simulink model "w3_warplab_trigger_proc"  (Simulink 7.7)
settings: Solver=ode45  StartTime=0.0  StopTime=100  RelTol=1e-3
InitFcn:
  | warplab_trigger_proc_init
StartFcn:
  | warplab_trigger_proc_init
undefined symbols (not defined in the file or in its folder): gcbh, xlBlockLoadCallback, xlGetNormalizedPeriod
libraries: xbsIndex_r4 x817, xbsEDKLib_r4 x1
(part 4 of 6)

== system w3_warplab_trigger_proc/Registers/Input Configuration Slice2 ==
  32b : Inport
  (LSB+0):(LSB+4) : xbsIndex_r4/Slice  nbits=5  boolean_output=off  mode=Lower Bit Location + Width  bit1=0  base1=MSB of Input  bit0=0  base0=LSB of Input  dbl_ovrd=off  block_type=slice
  (LSB+16):(LSB+20) : xbsIndex_r4/Slice  nbits=5  boolean_output=off  mode=Lower Bit Location + Width  bit1=0  base1=MSB of Input  bit0=16  base0=LSB of Input  dbl_ovrd=off  block_type=slice
  (LSB+24):(LSB+28) : xbsIndex_r4/Slice  nbits=5  boolean_output=off  mode=Lower Bit Location + Width  bit1=0  base1=MSB of Input  bit0=24  base0=LSB of Input  dbl_ovrd=off  block_type=slice
  (LSB+8):(LSB+12) : xbsIndex_r4/Slice  nbits=5  boolean_output=off  mode=Lower Bit Location + Width  bit1=0  base1=MSB of Input  bit0=8  base0=LSB of Input  dbl_ovrd=off  block_type=slice
  LSB+13 : xbsIndex_r4/Slice  nbits=1  boolean_output=off  mode=Lower Bit Location + Width  bit1=0  base1=MSB of Input  bit0=13  base0=LSB of Input  dbl_ovrd=off  block_type=slice
  LSB+14 : xbsIndex_r4/Slice  nbits=1  boolean_output=off  mode=Lower Bit Location + Width  bit1=0  base1=MSB of Input  bit0=14  base0=LSB of Input  dbl_ovrd=off  block_type=slice
  LSB+21 : xbsIndex_r4/Slice  nbits=1  boolean_output=off  mode=Lower Bit Location + Width  bit1=0  base1=MSB of Input  bit0=21  base0=LSB of Input  dbl_ovrd=off  block_type=slice
  LSB+22 : xbsIndex_r4/Slice  nbits=1  boolean_output=off  mode=Lower Bit Location + Width  bit1=0  base1=MSB of Input  bit0=22  base0=LSB of Input  dbl_ovrd=off  block_type=slice
  LSB+29 : xbsIndex_r4/Slice  nbits=1  boolean_output=off  mode=Lower Bit Location + Width  bit1=0  base1=MSB of Input  bit0=29  base0=LSB of Input  dbl_ovrd=off  block_type=slice
  LSB+31 : xbsIndex_r4/Slice  nbits=1  boolean_output=off  mode=Lower Bit Location + Width  bit1=0  base1=MSB of Input  bit0=31  base0=LSB of Input  dbl_ovrd=off  block_type=slice
  LSB+5 : xbsIndex_r4/Slice  nbits=1  boolean_output=off  mode=Lower Bit Location + Width  bit1=0  base1=MSB of Input  bit0=5  base0=LSB of Input  dbl_ovrd=off  block_type=slice
  LSB+6 : xbsIndex_r4/Slice  nbits=1  boolean_output=off  mode=Lower Bit Location + Width  bit1=0  base1=MSB of Input  bit0=6  base0=LSB of Input  dbl_ovrd=off  block_type=slice
  Delay 1 : Outport
  Debounce 1 : Outport  Port=2
  Reset 1 : Outport  Port=3
  Delay 2 : Outport  Port=4
  Debounce 2 : Outport  Port=5
  Reset 2 : Outport  Port=6
  Delay 3 : Outport  Port=7
  Debounce 3 : Outport  Port=8
  Reset 3 : Outport  Port=9
  Delay 4 : Outport  Port=10
  Soft Trig : Outport  Port=11
  Reset 4 : Outport  Port=12
  wires:
  LSB+31/1 -> Reset 4/1
  LSB+29/1 -> Soft Trig/1
  (LSB+24):(LSB+28)/1 -> Delay 4/1
  LSB+22/1 -> Reset 3/1
  LSB+21/1 -> Debounce 3/1
  (LSB+16):(LSB+20)/1 -> Delay 3/1
  LSB+14/1 -> Reset 2/1
  LSB+13/1 -> Debounce 2/1
  (LSB+8):(LSB+12)/1 -> Delay 2/1
  LSB+6/1 -> Reset 1/1
  LSB+5/1 -> Debounce 1/1
  (LSB+0):(LSB+4)/1 -> Delay 1/1
  32b/1 -> (LSB+0):(LSB+4)/1, LSB+5/1, LSB+6/1, (LSB+8):(LSB+12)/1, LSB+13/1, LSB+14/1, (LSB+16):(LSB+20)/1, LSB+21/1, LSB+22/1, (LSB+24):(LSB+28)/1, LSB+29/1, LSB+31/1

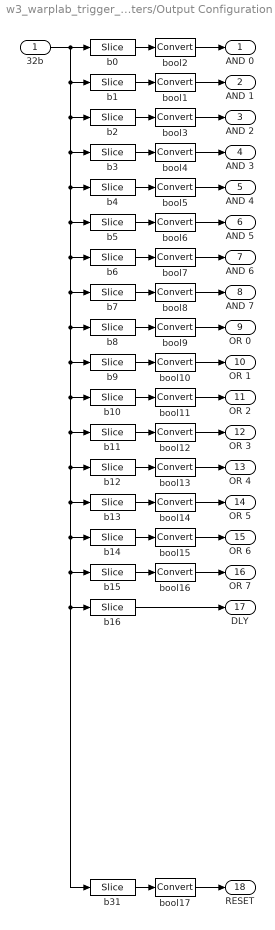
== system w3_warplab_trigger_proc/Registers/Output Configuration Slice ==
  32b : Inport
  b0 : xbsIndex_r4/Slice  nbits=1  boolean_output=off  mode=Lower Bit Location + Width  bit1=0  base1=MSB of Input  bit0=0  base0=LSB of Input  dbl_ovrd=off  block_type=slice
  b1 : xbsIndex_r4/Slice  nbits=1  boolean_output=off  mode=Lower Bit Location + Width  bit1=0  base1=MSB of Input  bit0=1  base0=LSB of Input  dbl_ovrd=off  block_type=slice
  b10 : xbsIndex_r4/Slice  nbits=1  boolean_output=off  mode=Lower Bit Location + Width  bit1=0  base1=MSB of Input  bit0=10  base0=LSB of Input  dbl_ovrd=off  block_type=slice
  b11 : xbsIndex_r4/Slice  nbits=1  boolean_output=off  mode=Lower Bit Location + Width  bit1=0  base1=MSB of Input  bit0=11  base0=LSB of Input  dbl_ovrd=off  block_type=slice
  b12 : xbsIndex_r4/Slice  nbits=1  boolean_output=off  mode=Lower Bit Location + Width  bit1=0  base1=MSB of Input  bit0=12  base0=LSB of Input  dbl_ovrd=off  block_type=slice
  b13 : xbsIndex_r4/Slice  nbits=1  boolean_output=off  mode=Lower Bit Location + Width  bit1=0  base1=MSB of Input  bit0=13  base0=LSB of Input  dbl_ovrd=off  block_type=slice
  b14 : xbsIndex_r4/Slice  nbits=1  boolean_output=off  mode=Lower Bit Location + Width  bit1=0  base1=MSB of Input  bit0=14  base0=LSB of Input  dbl_ovrd=off  block_type=slice
  b15 : xbsIndex_r4/Slice  nbits=1  boolean_output=off  mode=Lower Bit Location + Width  bit1=0  base1=MSB of Input  bit0=15  base0=LSB of Input  dbl_ovrd=off  block_type=slice
  b16 : xbsIndex_r4/Slice  nbits=5  boolean_output=off  mode=Lower Bit Location + Width  bit1=0  base1=MSB of Input  bit0=16  base0=LSB of Input  dbl_ovrd=off  block_type=slice
  b2 : xbsIndex_r4/Slice  nbits=1  boolean_output=off  mode=Lower Bit Location + Width  bit1=0  base1=MSB of Input  bit0=2  base0=LSB of Input  dbl_ovrd=off  block_type=slice
  b3 : xbsIndex_r4/Slice  nbits=1  boolean_output=off  mode=Lower Bit Location + Width  bit1=0  base1=MSB of Input  bit0=3  base0=LSB of Input  dbl_ovrd=off  block_type=slice
  b31 : xbsIndex_r4/Slice  nbits=1  boolean_output=off  mode=Lower Bit Location + Width  bit1=0  base1=MSB of Input  bit0=31  base0=LSB of Input  dbl_ovrd=off  block_type=slice
  b4 : xbsIndex_r4/Slice  nbits=1  boolean_output=off  mode=Lower Bit Location + Width  bit1=0  base1=MSB of Input  bit0=4  base0=LSB of Input  dbl_ovrd=off  block_type=slice
  b5 : xbsIndex_r4/Slice  nbits=1  boolean_output=off  mode=Lower Bit Location + Width  bit1=0  base1=MSB of Input  bit0=5  base0=LSB of Input  dbl_ovrd=off  block_type=slice
  b6 : xbsIndex_r4/Slice  nbits=1  boolean_output=off  mode=Lower Bit Location + Width  bit1=0  base1=MSB of Input  bit0=6  base0=LSB of Input  dbl_ovrd=off  block_type=slice
  b7 : xbsIndex_r4/Slice  nbits=1  boolean_output=off  mode=Lower Bit Location + Width  bit1=0  base1=MSB of Input  bit0=7  base0=LSB of Input  dbl_ovrd=off  block_type=slice
  b8 : xbsIndex_r4/Slice  nbits=1  boolean_output=off  mode=Lower Bit Location + Width  bit1=0  base1=MSB of Input  bit0=8  base0=LSB of Input  dbl_ovrd=off  block_type=slice
  b9 : xbsIndex_r4/Slice  nbits=1  boolean_output=off  mode=Lower Bit Location + Width  bit1=0  base1=MSB of Input  bit0=9  base0=LSB of Input  dbl_ovrd=off  block_type=slice
  bool{1..17} (17 alike) : xbsIndex_r4/Convert  gui_display_data_type=Boolean  arith_type=Boolean  n_bits=16  bin_pt=14  float_type=Single  exp_bits=8  fraction_bits=24  quantization=Truncate  overflow=Wrap  en=off  latency=0  dbl_ovrd=off  pipeline=off  block_type=convert
  AND 0 : Outport
  AND 1 : Outport  Port=2
  AND 2 : Outport  Port=3
  AND 3 : Outport  Port=4
  AND 4 : Outport  Port=5
  AND 5 : Outport  Port=6
  AND 6 : Outport  Port=7
  AND 7 : Outport  Port=8
  OR 0 : Outport  Port=9
  OR 1 : Outport  Port=10
  OR 2 : Outport  Port=11
  OR 3 : Outport  Port=12
  OR 4 : Outport  Port=13
  OR 5 : Outport  Port=14
  OR 6 : Outport  Port=15
  OR 7 : Outport  Port=16
  DLY : Outport  Port=17
  RESET : Outport  Port=18
  wires:
  32b/1 -> b0/1, b1/1, b2/1, b3/1, b4/1, b5/1, b6/1, b7/1, b8/1, b9/1, b10/1, b11/1, b12/1, b13/1, b14/1, b15/1, b31/1, b16/1
  b0/1 -> bool2/1
  b1/1 -> bool1/1
  b2/1 -> bool3/1
  b3/1 -> bool4/1
  b4/1 -> bool5/1
  b5/1 -> bool6/1
  b6/1 -> bool7/1
  b7/1 -> bool8/1
  b8/1 -> bool9/1
  b9/1 -> bool10/1
  b10/1 -> bool11/1
  b11/1 -> bool12/1
  b12/1 -> bool13/1
  b13/1 -> bool14/1
  b14/1 -> bool15/1
  b31/1 -> bool17/1
  b15/1 -> bool16/1
  bool2/1 -> AND 0/1
  bool1/1 -> AND 1/1
  bool3/1 -> AND 2/1
  bool4/1 -> AND 3/1
  bool5/1 -> AND 4/1
  bool6/1 -> AND 5/1
  bool7/1 -> AND 6/1
  bool8/1 -> AND 7/1
  bool9/1 -> OR 0/1
  bool10/1 -> OR 1/1
  bool11/1 -> OR 2/1
  bool12/1 -> OR 3/1
  bool13/1 -> OR 4/1
  bool14/1 -> OR 5/1
  bool15/1 -> OR 6/1
  bool16/1 -> OR 7/1
  bool17/1 -> RESET/1
  b16/1 -> DLY/1

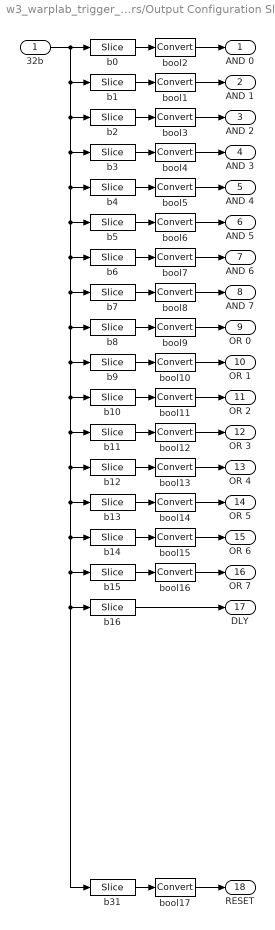
== system w3_warplab_trigger_proc/Registers/Output Configuration Slice1 ==
  32b : Inport
  b0 : xbsIndex_r4/Slice  nbits=1  boolean_output=off  mode=Lower Bit Location + Width  bit1=0  base1=MSB of Input  bit0=0  base0=LSB of Input  dbl_ovrd=off  block_type=slice
  b1 : xbsIndex_r4/Slice  nbits=1  boolean_output=off  mode=Lower Bit Location + Width  bit1=0  base1=MSB of Input  bit0=1  base0=LSB of Input  dbl_ovrd=off  block_type=slice
  b10 : xbsIndex_r4/Slice  nbits=1  boolean_output=off  mode=Lower Bit Location + Width  bit1=0  base1=MSB of Input  bit0=10  base0=LSB of Input  dbl_ovrd=off  block_type=slice
  b11 : xbsIndex_r4/Slice  nbits=1  boolean_output=off  mode=Lower Bit Location + Width  bit1=0  base1=MSB of Input  bit0=11  base0=LSB of Input  dbl_ovrd=off  block_type=slice
  b12 : xbsIndex_r4/Slice  nbits=1  boolean_output=off  mode=Lower Bit Location + Width  bit1=0  base1=MSB of Input  bit0=12  base0=LSB of Input  dbl_ovrd=off  block_type=slice
  b13 : xbsIndex_r4/Slice  nbits=1  boolean_output=off  mode=Lower Bit Location + Width  bit1=0  base1=MSB of Input  bit0=13  base0=LSB of Input  dbl_ovrd=off  block_type=slice
  b14 : xbsIndex_r4/Slice  nbits=1  boolean_output=off  mode=Lower Bit Location + Width  bit1=0  base1=MSB of Input  bit0=14  base0=LSB of Input  dbl_ovrd=off  block_type=slice
  b15 : xbsIndex_r4/Slice  nbits=1  boolean_output=off  mode=Lower Bit Location + Width  bit1=0  base1=MSB of Input  bit0=15  base0=LSB of Input  dbl_ovrd=off  block_type=slice
  b16 : xbsIndex_r4/Slice  nbits=5  boolean_output=off  mode=Lower Bit Location + Width  bit1=0  base1=MSB of Input  bit0=16  base0=LSB of Input  dbl_ovrd=off  block_type=slice
  b2 : xbsIndex_r4/Slice  nbits=1  boolean_output=off  mode=Lower Bit Location + Width  bit1=0  base1=MSB of Input  bit0=2  base0=LSB of Input  dbl_ovrd=off  block_type=slice
  b3 : xbsIndex_r4/Slice  nbits=1  boolean_output=off  mode=Lower Bit Location + Width  bit1=0  base1=MSB of Input  bit0=3  base0=LSB of Input  dbl_ovrd=off  block_type=slice
  b31 : xbsIndex_r4/Slice  nbits=1  boolean_output=off  mode=Lower Bit Location + Width  bit1=0  base1=MSB of Input  bit0=31  base0=LSB of Input  dbl_ovrd=off  block_type=slice
  b4 : xbsIndex_r4/Slice  nbits=1  boolean_output=off  mode=Lower Bit Location + Width  bit1=0  base1=MSB of Input  bit0=4  base0=LSB of Input  dbl_ovrd=off  block_type=slice
  b5 : xbsIndex_r4/Slice  nbits=1  boolean_output=off  mode=Lower Bit Location + Width  bit1=0  base1=MSB of Input  bit0=5  base0=LSB of Input  dbl_ovrd=off  block_type=slice
  b6 : xbsIndex_r4/Slice  nbits=1  boolean_output=off  mode=Lower Bit Location + Width  bit1=0  base1=MSB of Input  bit0=6  base0=LSB of Input  dbl_ovrd=off  block_type=slice
  b7 : xbsIndex_r4/Slice  nbits=1  boolean_output=off  mode=Lower Bit Location + Width  bit1=0  base1=MSB of Input  bit0=7  base0=LSB of Input  dbl_ovrd=off  block_type=slice
  b8 : xbsIndex_r4/Slice  nbits=1  boolean_output=off  mode=Lower Bit Location + Width  bit1=0  base1=MSB of Input  bit0=8  base0=LSB of Input  dbl_ovrd=off  block_type=slice
  b9 : xbsIndex_r4/Slice  nbits=1  boolean_output=off  mode=Lower Bit Location + Width  bit1=0  base1=MSB of Input  bit0=9  base0=LSB of Input  dbl_ovrd=off  block_type=slice
  bool{1..17} (17 alike) : xbsIndex_r4/Convert  gui_display_data_type=Boolean  arith_type=Boolean  n_bits=16  bin_pt=14  float_type=Single  exp_bits=8  fraction_bits=24  quantization=Truncate  overflow=Wrap  en=off  latency=0  dbl_ovrd=off  pipeline=off  block_type=convert
  AND 0 : Outport
  AND 1 : Outport  Port=2
  AND 2 : Outport  Port=3
  AND 3 : Outport  Port=4
  AND 4 : Outport  Port=5
  AND 5 : Outport  Port=6
  AND 6 : Outport  Port=7
  AND 7 : Outport  Port=8
  OR 0 : Outport  Port=9
  OR 1 : Outport  Port=10
  OR 2 : Outport  Port=11
  OR 3 : Outport  Port=12
  OR 4 : Outport  Port=13
  OR 5 : Outport  Port=14
  OR 6 : Outport  Port=15
  OR 7 : Outport  Port=16
  DLY : Outport  Port=17
  RESET : Outport  Port=18
  wires:
  b16/1 -> DLY/1
  bool17/1 -> RESET/1
  bool16/1 -> OR 7/1
  bool15/1 -> OR 6/1
  bool14/1 -> OR 5/1
  bool13/1 -> OR 4/1
  bool12/1 -> OR 3/1
  bool11/1 -> OR 2/1
  bool10/1 -> OR 1/1
  bool9/1 -> OR 0/1
  bool8/1 -> AND 7/1
  bool7/1 -> AND 6/1
  bool6/1 -> AND 5/1
  bool5/1 -> AND 4/1
  bool4/1 -> AND 3/1
  bool3/1 -> AND 2/1
  bool1/1 -> AND 1/1
  bool2/1 -> AND 0/1
  b15/1 -> bool16/1
  b31/1 -> bool17/1
  b14/1 -> bool15/1
  b13/1 -> bool14/1
  b12/1 -> bool13/1
  b11/1 -> bool12/1
  b10/1 -> bool11/1
  b9/1 -> bool10/1
  b8/1 -> bool9/1
  b7/1 -> bool8/1
  b6/1 -> bool7/1
  b5/1 -> bool6/1
  b4/1 -> bool5/1
  b3/1 -> bool4/1
  b2/1 -> bool3/1
  b1/1 -> bool1/1
  b0/1 -> bool2/1
  32b/1 -> b16/1, b31/1, b15/1, b14/1, b13/1, b12/1, b11/1, b10/1, b9/1, b8/1, b7/1, b6/1, b5/1, b4/1, b3/1, b2/1, b1/1, b0/1

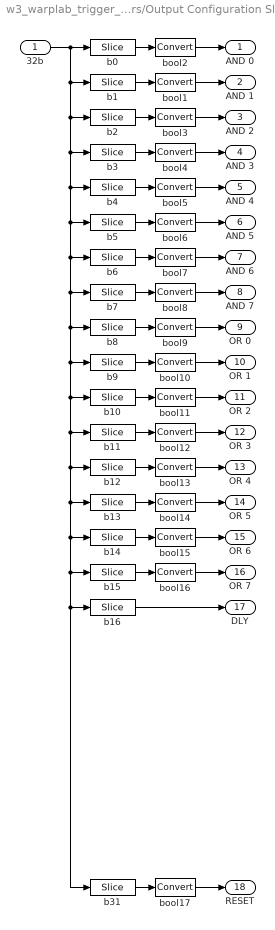
== system w3_warplab_trigger_proc/Registers/Output Configuration Slice2 ==
  32b : Inport
  b0 : xbsIndex_r4/Slice  nbits=1  boolean_output=off  mode=Lower Bit Location + Width  bit1=0  base1=MSB of Input  bit0=0  base0=LSB of Input  dbl_ovrd=off  block_type=slice
  b1 : xbsIndex_r4/Slice  nbits=1  boolean_output=off  mode=Lower Bit Location + Width  bit1=0  base1=MSB of Input  bit0=1  base0=LSB of Input  dbl_ovrd=off  block_type=slice
  b10 : xbsIndex_r4/Slice  nbits=1  boolean_output=off  mode=Lower Bit Location + Width  bit1=0  base1=MSB of Input  bit0=10  base0=LSB of Input  dbl_ovrd=off  block_type=slice
  b11 : xbsIndex_r4/Slice  nbits=1  boolean_output=off  mode=Lower Bit Location + Width  bit1=0  base1=MSB of Input  bit0=11  base0=LSB of Input  dbl_ovrd=off  block_type=slice
  b12 : xbsIndex_r4/Slice  nbits=1  boolean_output=off  mode=Lower Bit Location + Width  bit1=0  base1=MSB of Input  bit0=12  base0=LSB of Input  dbl_ovrd=off  block_type=slice
  b13 : xbsIndex_r4/Slice  nbits=1  boolean_output=off  mode=Lower Bit Location + Width  bit1=0  base1=MSB of Input  bit0=13  base0=LSB of Input  dbl_ovrd=off  block_type=slice
  b14 : xbsIndex_r4/Slice  nbits=1  boolean_output=off  mode=Lower Bit Location + Width  bit1=0  base1=MSB of Input  bit0=14  base0=LSB of Input  dbl_ovrd=off  block_type=slice
  b15 : xbsIndex_r4/Slice  nbits=1  boolean_output=off  mode=Lower Bit Location + Width  bit1=0  base1=MSB of Input  bit0=15  base0=LSB of Input  dbl_ovrd=off  block_type=slice
  b16 : xbsIndex_r4/Slice  nbits=5  boolean_output=off  mode=Lower Bit Location + Width  bit1=0  base1=MSB of Input  bit0=16  base0=LSB of Input  dbl_ovrd=off  block_type=slice
  b2 : xbsIndex_r4/Slice  nbits=1  boolean_output=off  mode=Lower Bit Location + Width  bit1=0  base1=MSB of Input  bit0=2  base0=LSB of Input  dbl_ovrd=off  block_type=slice
  b3 : xbsIndex_r4/Slice  nbits=1  boolean_output=off  mode=Lower Bit Location + Width  bit1=0  base1=MSB of Input  bit0=3  base0=LSB of Input  dbl_ovrd=off  block_type=slice
  b31 : xbsIndex_r4/Slice  nbits=1  boolean_output=off  mode=Lower Bit Location + Width  bit1=0  base1=MSB of Input  bit0=31  base0=LSB of Input  dbl_ovrd=off  block_type=slice
  b4 : xbsIndex_r4/Slice  nbits=1  boolean_output=off  mode=Lower Bit Location + Width  bit1=0  base1=MSB of Input  bit0=4  base0=LSB of Input  dbl_ovrd=off  block_type=slice
  b5 : xbsIndex_r4/Slice  nbits=1  boolean_output=off  mode=Lower Bit Location + Width  bit1=0  base1=MSB of Input  bit0=5  base0=LSB of Input  dbl_ovrd=off  block_type=slice
  b6 : xbsIndex_r4/Slice  nbits=1  boolean_output=off  mode=Lower Bit Location + Width  bit1=0  base1=MSB of Input  bit0=6  base0=LSB of Input  dbl_ovrd=off  block_type=slice
  b7 : xbsIndex_r4/Slice  nbits=1  boolean_output=off  mode=Lower Bit Location + Width  bit1=0  base1=MSB of Input  bit0=7  base0=LSB of Input  dbl_ovrd=off  block_type=slice
  b8 : xbsIndex_r4/Slice  nbits=1  boolean_output=off  mode=Lower Bit Location + Width  bit1=0  base1=MSB of Input  bit0=8  base0=LSB of Input  dbl_ovrd=off  block_type=slice
  b9 : xbsIndex_r4/Slice  nbits=1  boolean_output=off  mode=Lower Bit Location + Width  bit1=0  base1=MSB of Input  bit0=9  base0=LSB of Input  dbl_ovrd=off  block_type=slice
  bool{1..17} (17 alike) : xbsIndex_r4/Convert  gui_display_data_type=Boolean  arith_type=Boolean  n_bits=16  bin_pt=14  float_type=Single  exp_bits=8  fraction_bits=24  quantization=Truncate  overflow=Wrap  en=off  latency=0  dbl_ovrd=off  pipeline=off  block_type=convert
  AND 0 : Outport
  AND 1 : Outport  Port=2
  AND 2 : Outport  Port=3
  AND 3 : Outport  Port=4
  AND 4 : Outport  Port=5
  AND 5 : Outport  Port=6
  AND 6 : Outport  Port=7
  AND 7 : Outport  Port=8
  OR 0 : Outport  Port=9
  OR 1 : Outport  Port=10
  OR 2 : Outport  Port=11
  OR 3 : Outport  Port=12
  OR 4 : Outport  Port=13
  OR 5 : Outport  Port=14
  OR 6 : Outport  Port=15
  OR 7 : Outport  Port=16
  DLY : Outport  Port=17
  RESET : Outport  Port=18
  wires:
  32b/1 -> b0/1, b1/1, b2/1, b3/1, b4/1, b5/1, b6/1, b7/1, b8/1, b9/1, b10/1, b11/1, b12/1, b13/1, b14/1, b15/1, b31/1, b16/1
  b0/1 -> bool2/1
  b1/1 -> bool1/1
  b2/1 -> bool3/1
  b3/1 -> bool4/1
  b4/1 -> bool5/1
  b5/1 -> bool6/1
  b6/1 -> bool7/1
  b7/1 -> bool8/1
  b8/1 -> bool9/1
  b9/1 -> bool10/1
  b10/1 -> bool11/1
  b11/1 -> bool12/1
  b12/1 -> bool13/1
  b13/1 -> bool14/1
  b14/1 -> bool15/1
  b31/1 -> bool17/1
  b15/1 -> bool16/1
  bool2/1 -> AND 0/1
  bool1/1 -> AND 1/1
  bool3/1 -> AND 2/1
  bool4/1 -> AND 3/1
  bool5/1 -> AND 4/1
  bool6/1 -> AND 5/1
  bool7/1 -> AND 6/1
  bool8/1 -> AND 7/1
  bool9/1 -> OR 0/1
  bool10/1 -> OR 1/1
  bool11/1 -> OR 2/1
  bool12/1 -> OR 3/1
  bool13/1 -> OR 4/1
  bool14/1 -> OR 5/1
  bool15/1 -> OR 6/1
  bool16/1 -> OR 7/1
  bool17/1 -> RESET/1
  b16/1 -> DLY/1

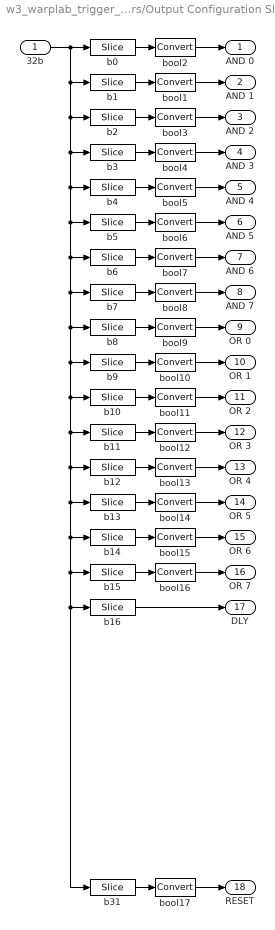
== system w3_warplab_trigger_proc/Registers/Output Configuration Slice3 ==
  32b : Inport
  b0 : xbsIndex_r4/Slice  nbits=1  boolean_output=off  mode=Lower Bit Location + Width  bit1=0  base1=MSB of Input  bit0=0  base0=LSB of Input  dbl_ovrd=off  block_type=slice
  b1 : xbsIndex_r4/Slice  nbits=1  boolean_output=off  mode=Lower Bit Location + Width  bit1=0  base1=MSB of Input  bit0=1  base0=LSB of Input  dbl_ovrd=off  block_type=slice
  b10 : xbsIndex_r4/Slice  nbits=1  boolean_output=off  mode=Lower Bit Location + Width  bit1=0  base1=MSB of Input  bit0=10  base0=LSB of Input  dbl_ovrd=off  block_type=slice
  b11 : xbsIndex_r4/Slice  nbits=1  boolean_output=off  mode=Lower Bit Location + Width  bit1=0  base1=MSB of Input  bit0=11  base0=LSB of Input  dbl_ovrd=off  block_type=slice
  b12 : xbsIndex_r4/Slice  nbits=1  boolean_output=off  mode=Lower Bit Location + Width  bit1=0  base1=MSB of Input  bit0=12  base0=LSB of Input  dbl_ovrd=off  block_type=slice
  b13 : xbsIndex_r4/Slice  nbits=1  boolean_output=off  mode=Lower Bit Location + Width  bit1=0  base1=MSB of Input  bit0=13  base0=LSB of Input  dbl_ovrd=off  block_type=slice
  b14 : xbsIndex_r4/Slice  nbits=1  boolean_output=off  mode=Lower Bit Location + Width  bit1=0  base1=MSB of Input  bit0=14  base0=LSB of Input  dbl_ovrd=off  block_type=slice
  b15 : xbsIndex_r4/Slice  nbits=1  boolean_output=off  mode=Lower Bit Location + Width  bit1=0  base1=MSB of Input  bit0=15  base0=LSB of Input  dbl_ovrd=off  block_type=slice
  b16 : xbsIndex_r4/Slice  nbits=5  boolean_output=off  mode=Lower Bit Location + Width  bit1=0  base1=MSB of Input  bit0=16  base0=LSB of Input  dbl_ovrd=off  block_type=slice
  b2 : xbsIndex_r4/Slice  nbits=1  boolean_output=off  mode=Lower Bit Location + Width  bit1=0  base1=MSB of Input  bit0=2  base0=LSB of Input  dbl_ovrd=off  block_type=slice
  b3 : xbsIndex_r4/Slice  nbits=1  boolean_output=off  mode=Lower Bit Location + Width  bit1=0  base1=MSB of Input  bit0=3  base0=LSB of Input  dbl_ovrd=off  block_type=slice
  b31 : xbsIndex_r4/Slice  nbits=1  boolean_output=off  mode=Lower Bit Location + Width  bit1=0  base1=MSB of Input  bit0=31  base0=LSB of Input  dbl_ovrd=off  block_type=slice
  b4 : xbsIndex_r4/Slice  nbits=1  boolean_output=off  mode=Lower Bit Location + Width  bit1=0  base1=MSB of Input  bit0=4  base0=LSB of Input  dbl_ovrd=off  block_type=slice
  b5 : xbsIndex_r4/Slice  nbits=1  boolean_output=off  mode=Lower Bit Location + Width  bit1=0  base1=MSB of Input  bit0=5  base0=LSB of Input  dbl_ovrd=off  block_type=slice
  b6 : xbsIndex_r4/Slice  nbits=1  boolean_output=off  mode=Lower Bit Location + Width  bit1=0  base1=MSB of Input  bit0=6  base0=LSB of Input  dbl_ovrd=off  block_type=slice
  b7 : xbsIndex_r4/Slice  nbits=1  boolean_output=off  mode=Lower Bit Location + Width  bit1=0  base1=MSB of Input  bit0=7  base0=LSB of Input  dbl_ovrd=off  block_type=slice
  b8 : xbsIndex_r4/Slice  nbits=1  boolean_output=off  mode=Lower Bit Location + Width  bit1=0  base1=MSB of Input  bit0=8  base0=LSB of Input  dbl_ovrd=off  block_type=slice
  b9 : xbsIndex_r4/Slice  nbits=1  boolean_output=off  mode=Lower Bit Location + Width  bit1=0  base1=MSB of Input  bit0=9  base0=LSB of Input  dbl_ovrd=off  block_type=slice
  bool{1..17} (17 alike) : xbsIndex_r4/Convert  gui_display_data_type=Boolean  arith_type=Boolean  n_bits=16  bin_pt=14  float_type=Single  exp_bits=8  fraction_bits=24  quantization=Truncate  overflow=Wrap  en=off  latency=0  dbl_ovrd=off  pipeline=off  block_type=convert
  AND 0 : Outport
  AND 1 : Outport  Port=2
  AND 2 : Outport  Port=3
  AND 3 : Outport  Port=4
  AND 4 : Outport  Port=5
  AND 5 : Outport  Port=6
  AND 6 : Outport  Port=7
  AND 7 : Outport  Port=8
  OR 0 : Outport  Port=9
  OR 1 : Outport  Port=10
  OR 2 : Outport  Port=11
  OR 3 : Outport  Port=12
  OR 4 : Outport  Port=13
  OR 5 : Outport  Port=14
  OR 6 : Outport  Port=15
  OR 7 : Outport  Port=16
  DLY : Outport  Port=17
  RESET : Outport  Port=18
  wires:
  b16/1 -> DLY/1
  bool17/1 -> RESET/1
  bool16/1 -> OR 7/1
  bool15/1 -> OR 6/1
  bool14/1 -> OR 5/1
  bool13/1 -> OR 4/1
  bool12/1 -> OR 3/1
  bool11/1 -> OR 2/1
  bool10/1 -> OR 1/1
  bool9/1 -> OR 0/1
  bool8/1 -> AND 7/1
  bool7/1 -> AND 6/1
  bool6/1 -> AND 5/1
  bool5/1 -> AND 4/1
  bool4/1 -> AND 3/1
  bool3/1 -> AND 2/1
  bool1/1 -> AND 1/1
  bool2/1 -> AND 0/1
  b15/1 -> bool16/1
  b31/1 -> bool17/1
  b14/1 -> bool15/1
  b13/1 -> bool14/1
  b12/1 -> bool13/1
  b11/1 -> bool12/1
  b10/1 -> bool11/1
  b9/1 -> bool10/1
  b8/1 -> bool9/1
  b7/1 -> bool8/1
  b6/1 -> bool7/1
  b5/1 -> bool6/1
  b4/1 -> bool5/1
  b3/1 -> bool4/1
  b2/1 -> bool3/1
  b1/1 -> bool1/1
  b0/1 -> bool2/1
  32b/1 -> b16/1, b31/1, b15/1, b14/1, b13/1, b12/1, b11/1, b10/1, b9/1, b8/1, b7/1, b6/1, b5/1, b4/1, b3/1, b2/1, b1/1, b0/1

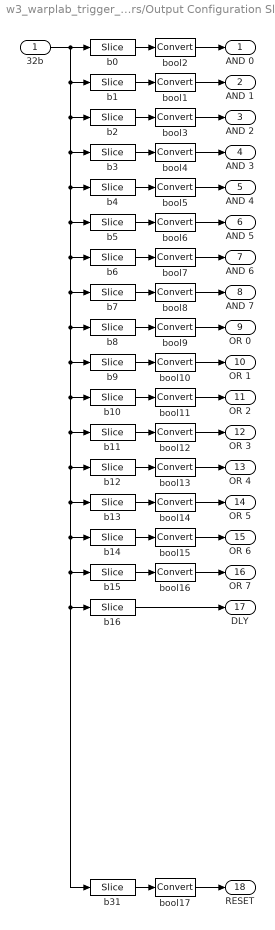
== system w3_warplab_trigger_proc/Registers/Output Configuration Slice4 ==
  32b : Inport
  b0 : xbsIndex_r4/Slice  nbits=1  boolean_output=off  mode=Lower Bit Location + Width  bit1=0  base1=MSB of Input  bit0=0  base0=LSB of Input  dbl_ovrd=off  block_type=slice
  b1 : xbsIndex_r4/Slice  nbits=1  boolean_output=off  mode=Lower Bit Location + Width  bit1=0  base1=MSB of Input  bit0=1  base0=LSB of Input  dbl_ovrd=off  block_type=slice
  b10 : xbsIndex_r4/Slice  nbits=1  boolean_output=off  mode=Lower Bit Location + Width  bit1=0  base1=MSB of Input  bit0=10  base0=LSB of Input  dbl_ovrd=off  block_type=slice
  b11 : xbsIndex_r4/Slice  nbits=1  boolean_output=off  mode=Lower Bit Location + Width  bit1=0  base1=MSB of Input  bit0=11  base0=LSB of Input  dbl_ovrd=off  block_type=slice
  b12 : xbsIndex_r4/Slice  nbits=1  boolean_output=off  mode=Lower Bit Location + Width  bit1=0  base1=MSB of Input  bit0=12  base0=LSB of Input  dbl_ovrd=off  block_type=slice
  b13 : xbsIndex_r4/Slice  nbits=1  boolean_output=off  mode=Lower Bit Location + Width  bit1=0  base1=MSB of Input  bit0=13  base0=LSB of Input  dbl_ovrd=off  block_type=slice
  b14 : xbsIndex_r4/Slice  nbits=1  boolean_output=off  mode=Lower Bit Location + Width  bit1=0  base1=MSB of Input  bit0=14  base0=LSB of Input  dbl_ovrd=off  block_type=slice
  b15 : xbsIndex_r4/Slice  nbits=1  boolean_output=off  mode=Lower Bit Location + Width  bit1=0  base1=MSB of Input  bit0=15  base0=LSB of Input  dbl_ovrd=off  block_type=slice
  b16 : xbsIndex_r4/Slice  nbits=5  boolean_output=off  mode=Lower Bit Location + Width  bit1=0  base1=MSB of Input  bit0=16  base0=LSB of Input  dbl_ovrd=off  block_type=slice
  b2 : xbsIndex_r4/Slice  nbits=1  boolean_output=off  mode=Lower Bit Location + Width  bit1=0  base1=MSB of Input  bit0=2  base0=LSB of Input  dbl_ovrd=off  block_type=slice
  b3 : xbsIndex_r4/Slice  nbits=1  boolean_output=off  mode=Lower Bit Location + Width  bit1=0  base1=MSB of Input  bit0=3  base0=LSB of Input  dbl_ovrd=off  block_type=slice
  b31 : xbsIndex_r4/Slice  nbits=1  boolean_output=off  mode=Lower Bit Location + Width  bit1=0  base1=MSB of Input  bit0=31  base0=LSB of Input  dbl_ovrd=off  block_type=slice
  b4 : xbsIndex_r4/Slice  nbits=1  boolean_output=off  mode=Lower Bit Location + Width  bit1=0  base1=MSB of Input  bit0=4  base0=LSB of Input  dbl_ovrd=off  block_type=slice
  b5 : xbsIndex_r4/Slice  nbits=1  boolean_output=off  mode=Lower Bit Location + Width  bit1=0  base1=MSB of Input  bit0=5  base0=LSB of Input  dbl_ovrd=off  block_type=slice
  b6 : xbsIndex_r4/Slice  nbits=1  boolean_output=off  mode=Lower Bit Location + Width  bit1=0  base1=MSB of Input  bit0=6  base0=LSB of Input  dbl_ovrd=off  block_type=slice
  b7 : xbsIndex_r4/Slice  nbits=1  boolean_output=off  mode=Lower Bit Location + Width  bit1=0  base1=MSB of Input  bit0=7  base0=LSB of Input  dbl_ovrd=off  block_type=slice
  b8 : xbsIndex_r4/Slice  nbits=1  boolean_output=off  mode=Lower Bit Location + Width  bit1=0  base1=MSB of Input  bit0=8  base0=LSB of Input  dbl_ovrd=off  block_type=slice
  b9 : xbsIndex_r4/Slice  nbits=1  boolean_output=off  mode=Lower Bit Location + Width  bit1=0  base1=MSB of Input  bit0=9  base0=LSB of Input  dbl_ovrd=off  block_type=slice
  bool{1..17} (17 alike) : xbsIndex_r4/Convert  gui_display_data_type=Boolean  arith_type=Boolean  n_bits=16  bin_pt=14  float_type=Single  exp_bits=8  fraction_bits=24  quantization=Truncate  overflow=Wrap  en=off  latency=0  dbl_ovrd=off  pipeline=off  block_type=convert
  AND 0 : Outport
  AND 1 : Outport  Port=2
  AND 2 : Outport  Port=3
  AND 3 : Outport  Port=4
  AND 4 : Outport  Port=5
  AND 5 : Outport  Port=6
  AND 6 : Outport  Port=7
  AND 7 : Outport  Port=8
  OR 0 : Outport  Port=9
  OR 1 : Outport  Port=10
  OR 2 : Outport  Port=11
  OR 3 : Outport  Port=12
  OR 4 : Outport  Port=13
  OR 5 : Outport  Port=14
  OR 6 : Outport  Port=15
  OR 7 : Outport  Port=16
  DLY : Outport  Port=17
  RESET : Outport  Port=18
  wires:
  32b/1 -> b0/1, b1/1, b2/1, b3/1, b4/1, b5/1, b6/1, b7/1, b8/1, b9/1, b10/1, b11/1, b12/1, b13/1, b14/1, b15/1, b31/1, b16/1
  b0/1 -> bool2/1
  b1/1 -> bool1/1
  b2/1 -> bool3/1
  b3/1 -> bool4/1
  b4/1 -> bool5/1
  b5/1 -> bool6/1
  b6/1 -> bool7/1
  b7/1 -> bool8/1
  b8/1 -> bool9/1
  b9/1 -> bool10/1
  b10/1 -> bool11/1
  b11/1 -> bool12/1
  b12/1 -> bool13/1
  b13/1 -> bool14/1
  b14/1 -> bool15/1
  b31/1 -> bool17/1
  b15/1 -> bool16/1
  bool2/1 -> AND 0/1
  bool1/1 -> AND 1/1
  bool3/1 -> AND 2/1
  bool4/1 -> AND 3/1
  bool5/1 -> AND 4/1
  bool6/1 -> AND 5/1
  bool7/1 -> AND 6/1
  bool8/1 -> AND 7/1
  bool9/1 -> OR 0/1
  bool10/1 -> OR 1/1
  bool11/1 -> OR 2/1
  bool12/1 -> OR 3/1
  bool13/1 -> OR 4/1
  bool14/1 -> OR 5/1
  bool15/1 -> OR 6/1
  bool16/1 -> OR 7/1
  bool17/1 -> RESET/1
  b16/1 -> DLY/1

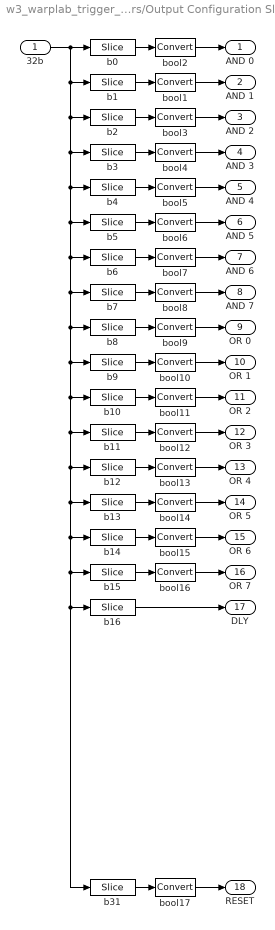
== system w3_warplab_trigger_proc/Registers/Output Configuration Slice5 ==
  32b : Inport
  b0 : xbsIndex_r4/Slice  nbits=1  boolean_output=off  mode=Lower Bit Location + Width  bit1=0  base1=MSB of Input  bit0=0  base0=LSB of Input  dbl_ovrd=off  block_type=slice
  b1 : xbsIndex_r4/Slice  nbits=1  boolean_output=off  mode=Lower Bit Location + Width  bit1=0  base1=MSB of Input  bit0=1  base0=LSB of Input  dbl_ovrd=off  block_type=slice
  b10 : xbsIndex_r4/Slice  nbits=1  boolean_output=off  mode=Lower Bit Location + Width  bit1=0  base1=MSB of Input  bit0=10  base0=LSB of Input  dbl_ovrd=off  block_type=slice
  b11 : xbsIndex_r4/Slice  nbits=1  boolean_output=off  mode=Lower Bit Location + Width  bit1=0  base1=MSB of Input  bit0=11  base0=LSB of Input  dbl_ovrd=off  block_type=slice
  b12 : xbsIndex_r4/Slice  nbits=1  boolean_output=off  mode=Lower Bit Location + Width  bit1=0  base1=MSB of Input  bit0=12  base0=LSB of Input  dbl_ovrd=off  block_type=slice
  b13 : xbsIndex_r4/Slice  nbits=1  boolean_output=off  mode=Lower Bit Location + Width  bit1=0  base1=MSB of Input  bit0=13  base0=LSB of Input  dbl_ovrd=off  block_type=slice
  b14 : xbsIndex_r4/Slice  nbits=1  boolean_output=off  mode=Lower Bit Location + Width  bit1=0  base1=MSB of Input  bit0=14  base0=LSB of Input  dbl_ovrd=off  block_type=slice
  b15 : xbsIndex_r4/Slice  nbits=1  boolean_output=off  mode=Lower Bit Location + Width  bit1=0  base1=MSB of Input  bit0=15  base0=LSB of Input  dbl_ovrd=off  block_type=slice
  b16 : xbsIndex_r4/Slice  nbits=5  boolean_output=off  mode=Lower Bit Location + Width  bit1=0  base1=MSB of Input  bit0=16  base0=LSB of Input  dbl_ovrd=off  block_type=slice
  b2 : xbsIndex_r4/Slice  nbits=1  boolean_output=off  mode=Lower Bit Location + Width  bit1=0  base1=MSB of Input  bit0=2  base0=LSB of Input  dbl_ovrd=off  block_type=slice
  b3 : xbsIndex_r4/Slice  nbits=1  boolean_output=off  mode=Lower Bit Location + Width  bit1=0  base1=MSB of Input  bit0=3  base0=LSB of Input  dbl_ovrd=off  block_type=slice
  b31 : xbsIndex_r4/Slice  nbits=1  boolean_output=off  mode=Lower Bit Location + Width  bit1=0  base1=MSB of Input  bit0=31  base0=LSB of Input  dbl_ovrd=off  block_type=slice
  b4 : xbsIndex_r4/Slice  nbits=1  boolean_output=off  mode=Lower Bit Location + Width  bit1=0  base1=MSB of Input  bit0=4  base0=LSB of Input  dbl_ovrd=off  block_type=slice
  b5 : xbsIndex_r4/Slice  nbits=1  boolean_output=off  mode=Lower Bit Location + Width  bit1=0  base1=MSB of Input  bit0=5  base0=LSB of Input  dbl_ovrd=off  block_type=slice
  b6 : xbsIndex_r4/Slice  nbits=1  boolean_output=off  mode=Lower Bit Location + Width  bit1=0  base1=MSB of Input  bit0=6  base0=LSB of Input  dbl_ovrd=off  block_type=slice
  b7 : xbsIndex_r4/Slice  nbits=1  boolean_output=off  mode=Lower Bit Location + Width  bit1=0  base1=MSB of Input  bit0=7  base0=LSB of Input  dbl_ovrd=off  block_type=slice
  b8 : xbsIndex_r4/Slice  nbits=1  boolean_output=off  mode=Lower Bit Location + Width  bit1=0  base1=MSB of Input  bit0=8  base0=LSB of Input  dbl_ovrd=off  block_type=slice
  b9 : xbsIndex_r4/Slice  nbits=1  boolean_output=off  mode=Lower Bit Location + Width  bit1=0  base1=MSB of Input  bit0=9  base0=LSB of Input  dbl_ovrd=off  block_type=slice
  bool{1..17} (17 alike) : xbsIndex_r4/Convert  gui_display_data_type=Boolean  arith_type=Boolean  n_bits=16  bin_pt=14  float_type=Single  exp_bits=8  fraction_bits=24  quantization=Truncate  overflow=Wrap  en=off  latency=0  dbl_ovrd=off  pipeline=off  block_type=convert
  AND 0 : Outport
  AND 1 : Outport  Port=2
  AND 2 : Outport  Port=3
  AND 3 : Outport  Port=4
  AND 4 : Outport  Port=5
  AND 5 : Outport  Port=6
  AND 6 : Outport  Port=7
  AND 7 : Outport  Port=8
  OR 0 : Outport  Port=9
  OR 1 : Outport  Port=10
  OR 2 : Outport  Port=11
  OR 3 : Outport  Port=12
  OR 4 : Outport  Port=13
  OR 5 : Outport  Port=14
  OR 6 : Outport  Port=15
  OR 7 : Outport  Port=16
  DLY : Outport  Port=17
  RESET : Outport  Port=18
  wires:
  b16/1 -> DLY/1
  bool17/1 -> RESET/1
  bool16/1 -> OR 7/1
  bool15/1 -> OR 6/1
  bool14/1 -> OR 5/1
  bool13/1 -> OR 4/1
  bool12/1 -> OR 3/1
  bool11/1 -> OR 2/1
  bool10/1 -> OR 1/1
  bool9/1 -> OR 0/1
  bool8/1 -> AND 7/1
  bool7/1 -> AND 6/1
  bool6/1 -> AND 5/1
  bool5/1 -> AND 4/1
  bool4/1 -> AND 3/1
  bool3/1 -> AND 2/1
  bool1/1 -> AND 1/1
  bool2/1 -> AND 0/1
  b15/1 -> bool16/1
  b31/1 -> bool17/1
  b14/1 -> bool15/1
  b13/1 -> bool14/1
  b12/1 -> bool13/1
  b11/1 -> bool12/1
  b10/1 -> bool11/1
  b9/1 -> bool10/1
  b8/1 -> bool9/1
  b7/1 -> bool8/1
  b6/1 -> bool7/1
  b5/1 -> bool6/1
  b4/1 -> bool5/1
  b3/1 -> bool4/1
  b2/1 -> bool3/1
  b1/1 -> bool1/1
  b0/1 -> bool2/1
  32b/1 -> b16/1, b31/1, b15/1, b14/1, b13/1, b12/1, b11/1, b10/1, b9/1, b8/1, b7/1, b6/1, b5/1, b4/1, b3/1, b2/1, b1/1, b0/1

== system w3_warplab_trigger_proc/Trigger Output 0/S-R Latch ==
  S : Inport
  R : Inport  Port=2
  Constant1 : xbsIndex_r4/Constant  const=1  gui_display_data_type=Fixed-point  arith_type=Unsigned  n_bits=1  bin_pt=0  preci_type=Single  exp_width=8  frac_width=24  explicit_period=off  period=1  equ=P=C  opselect=C  inp2=PCIN>>17  opr=+  inp1=P  carry=CIN  dbl_ovrd=off  block_type=constant
      settings: block_version=VER_STRING_GOES_HERE
  Convert1 : xbsIndex_r4/Convert  gui_display_data_type=Boolean  arith_type=Boolean  n_bits=16  bin_pt=14  float_type=Single  exp_bits=8  fraction_bits=24  quantization=Truncate  overflow=Wrap  en=off  latency=0  dbl_ovrd=off  pipeline=off  block_type=convert
  Convert2 : xbsIndex_r4/Convert  gui_display_data_type=Boolean  arith_type=Boolean  n_bits=16  bin_pt=14  float_type=Single  exp_bits=8  fraction_bits=24  quantization=Truncate  overflow=Wrap  en=off  latency=0  dbl_ovrd=off  pipeline=off  block_type=convert
  Register2 : xbsIndex_r4/Register  init=0  rst=on  en=on  dbl_ovrd=off  block_type=register
      settings: xl_area=[1 1 0 0 0 0 0]  block_version=VER_STRING_GOES_HERE
  Q : Outport
  wires:
  S/1 -> Convert2/1
  Register2/1 -> Q/1
  R/1 -> Convert1/1
  Constant1/1 -> Register2/1
  Convert1/1 -> Register2/2
  Convert2/1 -> Register2/3

== system w3_warplab_trigger_proc/Trigger Output 1/S-R Latch ==
  S : Inport
  R : Inport  Port=2
  Constant1 : xbsIndex_r4/Constant  const=1  gui_display_data_type=Fixed-point  arith_type=Unsigned  n_bits=1  bin_pt=0  preci_type=Single  exp_width=8  frac_width=24  explicit_period=off  period=1  equ=P=C  opselect=C  inp2=PCIN>>17  opr=+  inp1=P  carry=CIN  dbl_ovrd=off  block_type=constant
      settings: block_version=VER_STRING_GOES_HERE
  Convert1 : xbsIndex_r4/Convert  gui_display_data_type=Boolean  arith_type=Boolean  n_bits=16  bin_pt=14  float_type=Single  exp_bits=8  fraction_bits=24  quantization=Truncate  overflow=Wrap  en=off  latency=0  dbl_ovrd=off  pipeline=off  block_type=convert
  Convert2 : xbsIndex_r4/Convert  gui_display_data_type=Boolean  arith_type=Boolean  n_bits=16  bin_pt=14  float_type=Single  exp_bits=8  fraction_bits=24  quantization=Truncate  overflow=Wrap  en=off  latency=0  dbl_ovrd=off  pipeline=off  block_type=convert
  Register2 : xbsIndex_r4/Register  init=0  rst=on  en=on  dbl_ovrd=off  block_type=register
      settings: xl_area=[1 1 0 0 0 0 0]  block_version=VER_STRING_GOES_HERE
  Q : Outport
  wires:
  Convert2/1 -> Register2/3
  Convert1/1 -> Register2/2
  Constant1/1 -> Register2/1
  R/1 -> Convert1/1
  Register2/1 -> Q/1
  S/1 -> Convert2/1

== system w3_warplab_trigger_proc/Trigger Output 2/S-R Latch ==
  S : Inport
  R : Inport  Port=2
  Constant1 : xbsIndex_r4/Constant  const=1  gui_display_data_type=Fixed-point  arith_type=Unsigned  n_bits=1  bin_pt=0  preci_type=Single  exp_width=8  frac_width=24  explicit_period=off  period=1  equ=P=C  opselect=C  inp2=PCIN>>17  opr=+  inp1=P  carry=CIN  dbl_ovrd=off  block_type=constant
      settings: block_version=VER_STRING_GOES_HERE
  Convert1 : xbsIndex_r4/Convert  gui_display_data_type=Boolean  arith_type=Boolean  n_bits=16  bin_pt=14  float_type=Single  exp_bits=8  fraction_bits=24  quantization=Truncate  overflow=Wrap  en=off  latency=0  dbl_ovrd=off  pipeline=off  block_type=convert
  Convert2 : xbsIndex_r4/Convert  gui_display_data_type=Boolean  arith_type=Boolean  n_bits=16  bin_pt=14  float_type=Single  exp_bits=8  fraction_bits=24  quantization=Truncate  overflow=Wrap  en=off  latency=0  dbl_ovrd=off  pipeline=off  block_type=convert
  Register2 : xbsIndex_r4/Register  init=0  rst=on  en=on  dbl_ovrd=off  block_type=register
      settings: xl_area=[1 1 0 0 0 0 0]  block_version=VER_STRING_GOES_HERE
  Q : Outport
  wires:
  S/1 -> Convert2/1
  Register2/1 -> Q/1
  R/1 -> Convert1/1
  Constant1/1 -> Register2/1
  Convert1/1 -> Register2/2
  Convert2/1 -> Register2/3

== system w3_warplab_trigger_proc/Trigger Output 3/S-R Latch ==
  S : Inport
  R : Inport  Port=2
  Constant1 : xbsIndex_r4/Constant  const=1  gui_display_data_type=Fixed-point  arith_type=Unsigned  n_bits=1  bin_pt=0  preci_type=Single  exp_width=8  frac_width=24  explicit_period=off  period=1  equ=P=C  opselect=C  inp2=PCIN>>17  opr=+  inp1=P  carry=CIN  dbl_ovrd=off  block_type=constant
      settings: block_version=VER_STRING_GOES_HERE
  Convert1 : xbsIndex_r4/Convert  gui_display_data_type=Boolean  arith_type=Boolean  n_bits=16  bin_pt=14  float_type=Single  exp_bits=8  fraction_bits=24  quantization=Truncate  overflow=Wrap  en=off  latency=0  dbl_ovrd=off  pipeline=off  block_type=convert
  Convert2 : xbsIndex_r4/Convert  gui_display_data_type=Boolean  arith_type=Boolean  n_bits=16  bin_pt=14  float_type=Single  exp_bits=8  fraction_bits=24  quantization=Truncate  overflow=Wrap  en=off  latency=0  dbl_ovrd=off  pipeline=off  block_type=convert
  Register2 : xbsIndex_r4/Register  init=0  rst=on  en=on  dbl_ovrd=off  block_type=register
      settings: xl_area=[1 1 0 0 0 0 0]  block_version=VER_STRING_GOES_HERE
  Q : Outport
  wires:
  Convert2/1 -> Register2/3
  Convert1/1 -> Register2/2
  Constant1/1 -> Register2/1
  R/1 -> Convert1/1
  Register2/1 -> Q/1
  S/1 -> Convert2/1

== system w3_warplab_trigger_proc/Trigger Output 4/S-R Latch ==
  S : Inport
  R : Inport  Port=2
  Constant1 : xbsIndex_r4/Constant  const=1  gui_display_data_type=Fixed-point  arith_type=Unsigned  n_bits=1  bin_pt=0  preci_type=Single  exp_width=8  frac_width=24  explicit_period=off  period=1  equ=P=C  opselect=C  inp2=PCIN>>17  opr=+  inp1=P  carry=CIN  dbl_ovrd=off  block_type=constant
      settings: block_version=VER_STRING_GOES_HERE
  Convert1 : xbsIndex_r4/Convert  gui_display_data_type=Boolean  arith_type=Boolean  n_bits=16  bin_pt=14  float_type=Single  exp_bits=8  fraction_bits=24  quantization=Truncate  overflow=Wrap  en=off  latency=0  dbl_ovrd=off  pipeline=off  block_type=convert
  Convert2 : xbsIndex_r4/Convert  gui_display_data_type=Boolean  arith_type=Boolean  n_bits=16  bin_pt=14  float_type=Single  exp_bits=8  fraction_bits=24  quantization=Truncate  overflow=Wrap  en=off  latency=0  dbl_ovrd=off  pipeline=off  block_type=convert
  Register2 : xbsIndex_r4/Register  init=0  rst=on  en=on  dbl_ovrd=off  block_type=register
      settings: xl_area=[1 1 0 0 0 0 0]  block_version=VER_STRING_GOES_HERE
  Q : Outport
  wires:
  S/1 -> Convert2/1
  Register2/1 -> Q/1
  R/1 -> Convert1/1
  Constant1/1 -> Register2/1
  Convert1/1 -> Register2/2
  Convert2/1 -> Register2/3

== system w3_warplab_trigger_proc/Trigger Output 5/S-R Latch ==
  S : Inport
  R : Inport  Port=2
  Constant1 : xbsIndex_r4/Constant  const=1  gui_display_data_type=Fixed-point  arith_type=Unsigned  n_bits=1  bin_pt=0  preci_type=Single  exp_width=8  frac_width=24  explicit_period=off  period=1  equ=P=C  opselect=C  inp2=PCIN>>17  opr=+  inp1=P  carry=CIN  dbl_ovrd=off  block_type=constant
      settings: block_version=VER_STRING_GOES_HERE
  Convert1 : xbsIndex_r4/Convert  gui_display_data_type=Boolean  arith_type=Boolean  n_bits=16  bin_pt=14  float_type=Single  exp_bits=8  fraction_bits=24  quantization=Truncate  overflow=Wrap  en=off  latency=0  dbl_ovrd=off  pipeline=off  block_type=convert
  Convert2 : xbsIndex_r4/Convert  gui_display_data_type=Boolean  arith_type=Boolean  n_bits=16  bin_pt=14  float_type=Single  exp_bits=8  fraction_bits=24  quantization=Truncate  overflow=Wrap  en=off  latency=0  dbl_ovrd=off  pipeline=off  block_type=convert
  Register2 : xbsIndex_r4/Register  init=0  rst=on  en=on  dbl_ovrd=off  block_type=register
      settings: xl_area=[1 1 0 0 0 0 0]  block_version=VER_STRING_GOES_HERE
  Q : Outport
  wires:
  Convert2/1 -> Register2/3
  Convert1/1 -> Register2/2
  Constant1/1 -> Register2/1
  R/1 -> Convert1/1
  Register2/1 -> Q/1
  S/1 -> Convert2/1

== system w3_warplab_trigger_proc/Trigger Sources/AGC ==
  agc_done_in : xbsIndex_r4/Gateway In  gui_display_data_type=Boolean  arith_type=Boolean  n_bits=16  bin_pt=14  preci_type=Single  exp_width=8  frac_width=24  quantization="Round  (unbiased: +/- Inf)"  overflow=Saturate  period=1  dbl_ovrd=off  timing_constraint=None  locs_specified=off  LOCs={}  UseAsADC=off  ADCChannel='1'  inherit_from_input=off  hdl_port=on  block_type=gatewayin
  Trigger : Outport
  wires:
  agc_done_in/1 -> Trigger/1

== system w3_warplab_trigger_proc/Trigger Sources/Debug 0 ==
  Logical : xbsIndex_r4/Logical  logical_function=AND  inputs=4  en=off  latency=0  precision=Full  arith_type=Unsigned  n_bits=16  bin_pt=0  align_bp=on  dbl_ovrd=off  block_type=logical
  Mux : xbsIndex_r4/Mux  inputs=2  en=off  latency=0  precision=Full  arith_type=Unsigned  n_bits=16  bin_pt=14  quantization=Truncate  overflow=Wrap  dbl_ovrd=off  block_type=mux
  Register{,1..3} (4 alike) : xbsIndex_r4/Register  init=0  rst=off  en=off  dbl_ovrd=off  block_type=register
  Step : Step  Time=50  SampleTime=0
  debug_0_in : xbsIndex_r4/Gateway In  gui_display_data_type=Boolean  arith_type=Boolean  n_bits=16  bin_pt=14  preci_type=Single  exp_width=8  frac_width=24  quantization="Round  (unbiased: +/- Inf)"  overflow=Saturate  period=1  dbl_ovrd=off  timing_constraint=None  locs_specified=off  LOCs={}  UseAsADC=off  ADCChannel='1'  inherit_from_input=off  hdl_port=on  block_type=gatewayin
  Trigger : Outport
  wires:
  Mux/1 -> Trigger/1
  debug_0_in/1 -> Mux/2, Register/1
  Register/1 -> Register1/1, Logical/1
  Register1/1 -> Register2/1, Logical/2
  Register2/1 -> Register3/1, Logical/3
  [Debug_0_Debounce] -> Mux/1
  Register3/1 -> Logical/4
  Logical/1 -> Mux/3
  Step/1 -> debug_0_in/1

== system w3_warplab_trigger_proc/Trigger Sources/Debug 1 ==
  Logical : xbsIndex_r4/Logical  logical_function=AND  inputs=4  en=off  latency=0  precision=Full  arith_type=Unsigned  n_bits=16  bin_pt=0  align_bp=on  dbl_ovrd=off  block_type=logical
  Mux : xbsIndex_r4/Mux  inputs=2  en=off  latency=0  precision=Full  arith_type=Unsigned  n_bits=16  bin_pt=14  quantization=Truncate  overflow=Wrap  dbl_ovrd=off  block_type=mux
  Register{,1..3} (4 alike) : xbsIndex_r4/Register  init=0  rst=off  en=off  dbl_ovrd=off  block_type=register
  debug_1_in : xbsIndex_r4/Gateway In  gui_display_data_type=Boolean  arith_type=Boolean  n_bits=16  bin_pt=14  preci_type=Single  exp_width=8  frac_width=24  quantization="Round  (unbiased: +/- Inf)"  overflow=Saturate  period=1  dbl_ovrd=off  timing_constraint=None  locs_specified=off  LOCs={}  UseAsADC=off  ADCChannel='1'  inherit_from_input=off  hdl_port=on  block_type=gatewayin
  Trigger : Outport
  wires:
  Logical/1 -> Mux/3
  Register3/1 -> Logical/4
  [Debug_1_Debounce] -> Mux/1
  Register2/1 -> Logical/3, Register3/1
  Register1/1 -> Logical/2, Register2/1
  Register/1 -> Logical/1, Register1/1
  debug_1_in/1 -> Register/1, Mux/2
  Mux/1 -> Trigger/1

== system w3_warplab_trigger_proc/Trigger Sources/Debug 2 ==
  Logical : xbsIndex_r4/Logical  logical_function=AND  inputs=4  en=off  latency=0  precision=Full  arith_type=Unsigned  n_bits=16  bin_pt=0  align_bp=on  dbl_ovrd=off  block_type=logical
  Mux : xbsIndex_r4/Mux  inputs=2  en=off  latency=0  precision=Full  arith_type=Unsigned  n_bits=16  bin_pt=14  quantization=Truncate  overflow=Wrap  dbl_ovrd=off  block_type=mux
  Register{,1..3} (4 alike) : xbsIndex_r4/Register  init=0  rst=off  en=off  dbl_ovrd=off  block_type=register
  debug_2_in : xbsIndex_r4/Gateway In  gui_display_data_type=Boolean  arith_type=Boolean  n_bits=16  bin_pt=14  preci_type=Single  exp_width=8  frac_width=24  quantization="Round  (unbiased: +/- Inf)"  overflow=Saturate  period=1  dbl_ovrd=off  timing_constraint=None  locs_specified=off  LOCs={}  UseAsADC=off  ADCChannel='1'  inherit_from_input=off  hdl_port=on  block_type=gatewayin
  Trigger : Outport
  wires:
  Mux/1 -> Trigger/1
  debug_2_in/1 -> Mux/2, Register/1
  Register/1 -> Register1/1, Logical/1
  Register1/1 -> Register2/1, Logical/2
  Register2/1 -> Register3/1, Logical/3
  [Debug_2_Debounce] -> Mux/1
  Register3/1 -> Logical/4
  Logical/1 -> Mux/3

== system w3_warplab_trigger_proc/Trigger Sources/Debug 3 ==
  Logical : xbsIndex_r4/Logical  logical_function=AND  inputs=4  en=off  latency=0  precision=Full  arith_type=Unsigned  n_bits=16  bin_pt=0  align_bp=on  dbl_ovrd=off  block_type=logical
  Mux : xbsIndex_r4/Mux  inputs=2  en=off  latency=0  precision=Full  arith_type=Unsigned  n_bits=16  bin_pt=14  quantization=Truncate  overflow=Wrap  dbl_ovrd=off  block_type=mux
  Register{,1..3} (4 alike) : xbsIndex_r4/Register  init=0  rst=off  en=off  dbl_ovrd=off  block_type=register
  debug_3_in : xbsIndex_r4/Gateway In  gui_display_data_type=Boolean  arith_type=Boolean  n_bits=16  bin_pt=14  preci_type=Single  exp_width=8  frac_width=24  quantization="Round  (unbiased: +/- Inf)"  overflow=Saturate  period=1  dbl_ovrd=off  timing_constraint=None  locs_specified=off  LOCs={}  UseAsADC=off  ADCChannel='1'  inherit_from_input=off  hdl_port=on  block_type=gatewayin
  Trigger : Outport
  wires:
  Logical/1 -> Mux/3
  Register3/1 -> Logical/4
  [Debug_3_Debounce] -> Mux/1
  Register2/1 -> Logical/3, Register3/1
  Register1/1 -> Logical/2, Register2/1
  Register/1 -> Logical/1, Register1/1
  debug_3_in/1 -> Register/1, Mux/2
  Mux/1 -> Trigger/1
